simulink model "case4"  (R2024b)
settings: Solver=FixedStepAuto  StartTime=0  StopTime=1  FixedStep=1e-7  RelTol=1e-3
values from neighbouring files (symbols this model uses):
  SG_D_1_D = 0.01056    [IEEE9_case_parameters.m]    (also in case1_parameters.m; case2_parameters.m; case3_parameters.m; case4_parameters.m)
  SG_D_1_EnableSaturation = 0    [IEEE9_case_parameters.m]    (also in case1_parameters.m; case2_parameters.m; case3_parameters.m; case4_parameters.m)
  SG_D_1_f0 = 60    [IEEE9_case_parameters.m]    (also in case1_parameters.m; case2_parameters.m; case3_parameters.m; case4_parameters.m)
  SG_D_1_H = 7.5    [IEEE9_case_parameters.m]    (also in case1_parameters.m; case2_parameters.m; case3_parameters.m; case4_parameters.m)
  SG_D_1_K_A = 20    [IEEE9_case_parameters.m]    (also in case1_parameters.m; case2_parameters.m; case3_parameters.m; case4_parameters.m)
  SG_D_1_K_E = 1.000000e+1    (= 10)    [IEEE9_case_parameters.m]    (also in case1_parameters.m; case2_parameters.m; case3_parameters.m; case4_parameters.m)
  SG_D_1_K_F = 2.363    [IEEE9_case_parameters.m]    (also in case1_parameters.m; case2_parameters.m; case3_parameters.m; case4_parameters.m)
  SG_D_1_K_s = 0.5    [IEEE9_case_parameters.m]    (also in case1_parameters.m = 5; case2_parameters.m = 5; case3_parameters.m = 5; case4_parameters.m = 5)
  SG_D_1_R_a = 0.001088    [IEEE9_case_parameters.m]    (also in case1_parameters.m; case2_parameters.m; case3_parameters.m; case4_parameters.m)
  SG_D_1_S_A = 1    [IEEE9_case_parameters.m]    (also in case1_parameters.m; case2_parameters.m; case3_parameters.m; case4_parameters.m)
  SG_D_1_S_B = 0.103    [IEEE9_case_parameters.m]    (also in case1_parameters.m; case2_parameters.m; case3_parameters.m; case4_parameters.m)
  SG_D_1_S_N = 10.659857    [IEEE9_case_parameters.m]    (also in case1_parameters.m; case2_parameters.m; case3_parameters.m; case4_parameters.m)
  SG_D_1_SpeedPara = 200    [IEEE9_case_parameters.m]    (also in case1_parameters.m; case2_parameters.m; case3_parameters.m; case4_parameters.m)
  SG_D_1_T_0 = 0.720173    [IEEE9_case_parameters.m]    (also in case1_parameters.m = 0.755522; case2_parameters.m = 0.808931; case3_parameters.m = 0.869402; case4_parameters.m = 0.729316)
  SG_D_1_T_1 = 0.3    [IEEE9_case_parameters.m]    (also in case1_parameters.m; case2_parameters.m; case3_parameters.m; case4_parameters.m)
  SG_D_1_T_2 = 0.05    [IEEE9_case_parameters.m]    (also in case1_parameters.m; case2_parameters.m; case3_parameters.m; case4_parameters.m)
  SG_D_1_T_3 = 0.02    [IEEE9_case_parameters.m]    (also in case1_parameters.m; case2_parameters.m; case3_parameters.m; case4_parameters.m)
  SG_D_1_T_4 = 0.005    [IEEE9_case_parameters.m]    (also in case1_parameters.m; case2_parameters.m; case3_parameters.m; case4_parameters.m)
  SG_D_1_T_A = 0.02    [IEEE9_case_parameters.m]    (also in case1_parameters.m; case2_parameters.m; case3_parameters.m; case4_parameters.m)
  SG_D_1_T_dd = 8.000000e+0    (= 8)    [IEEE9_case_parameters.m]    (also in case1_parameters.m; case2_parameters.m; case3_parameters.m; case4_parameters.m)
  SG_D_1_T_ddd = 0.04    [IEEE9_case_parameters.m]    (also in case1_parameters.m; case2_parameters.m; case3_parameters.m; case4_parameters.m)
  SG_D_1_T_E = 0.314    [IEEE9_case_parameters.m]    (also in case1_parameters.m; case2_parameters.m; case3_parameters.m; case4_parameters.m)
  SG_D_1_T_F = 0.35    [IEEE9_case_parameters.m]    (also in case1_parameters.m; case2_parameters.m; case3_parameters.m; case4_parameters.m)
  SG_D_1_T_qd = 0.8    [IEEE9_case_parameters.m]    (also in case1_parameters.m; case2_parameters.m; case3_parameters.m; case4_parameters.m)
  SG_D_1_T_qdd = 0.02    [IEEE9_case_parameters.m]    (also in case1_parameters.m; case2_parameters.m; case3_parameters.m; case4_parameters.m)
  SG_D_1_T_speed = 0.1    [IEEE9_case_parameters.m]    (also in case1_parameters.m = 200; case2_parameters.m = 200; case3_parameters.m = 200; case4_parameters.m = 200)
  SG_D_1_T_w = 0.5    [IEEE9_case_parameters.m]    (also in case1_parameters.m; case2_parameters.m; case3_parameters.m; case4_parameters.m)
  SG_D_1_V_ref = 1.990276    [IEEE9_case_parameters.m]    (also in case1_parameters.m = 2.042296; case2_parameters.m = 2.051388; case3_parameters.m = 2.089584; case4_parameters.m = 2.01845)
  SG_D_1_w_ref = 376.991118    [IEEE9_case_parameters.m]    (also in case1_parameters.m; case2_parameters.m; case3_parameters.m; case4_parameters.m)
  SG_D_1_wb = 6.000000e+1    (= 60)    [IEEE9_case_parameters.m]    (also in case1_parameters.m; case2_parameters.m; case3_parameters.m; case4_parameters.m)
  SG_D_1_x_d = 1.9    [IEEE9_case_parameters.m]    (also in case1_parameters.m; case2_parameters.m; case3_parameters.m; case4_parameters.m)
  SG_D_1_x_dd = 0.302    [IEEE9_case_parameters.m]    (also in case1_parameters.m; case2_parameters.m; case3_parameters.m; case4_parameters.m)
  SG_D_1_x_ddd = 0.204    [IEEE9_case_parameters.m]    (also in case1_parameters.m; case2_parameters.m; case3_parameters.m; case4_parameters.m)
  SG_D_1_x_l = 0.05    [IEEE9_case_parameters.m]    (also in case1_parameters.m; case2_parameters.m; case3_parameters.m; case4_parameters.m)
  SG_D_1_x_q = 1.3    [IEEE9_case_parameters.m]    (also in case1_parameters.m; case2_parameters.m; case3_parameters.m; case4_parameters.m)
  SG_D_1_x_qd = 0.5    [IEEE9_case_parameters.m]    (also in case1_parameters.m; case2_parameters.m; case3_parameters.m; case4_parameters.m)
  SG_D_1_x_qdd = 0.3    [IEEE9_case_parameters.m]    (also in case1_parameters.m; case2_parameters.m; case3_parameters.m; case4_parameters.m)
  SG_D_2_D = 0.02    [IEEE9_case_parameters.m]    (also in case1_parameters.m; case2_parameters.m; case3_parameters.m; case4_parameters.m)
  SG_D_2_EnableSaturation = 0    [IEEE9_case_parameters.m]    (also in case1_parameters.m; case2_parameters.m; case3_parameters.m; case4_parameters.m)
  SG_D_2_f0 = 60    [IEEE9_case_parameters.m]    (also in case1_parameters.m; case2_parameters.m; case3_parameters.m; case4_parameters.m)
  SG_D_2_H = 8.000000e+0    (= 8)    [IEEE9_case_parameters.m]    (also in case1_parameters.m; case2_parameters.m; case3_parameters.m; case4_parameters.m)
  SG_D_2_K_A = 20    [IEEE9_case_parameters.m]    (also in case1_parameters.m; case2_parameters.m; case3_parameters.m; case4_parameters.m)
  SG_D_2_K_E = 1.000000e+1    (= 10)    [IEEE9_case_parameters.m]    (also in case1_parameters.m; case2_parameters.m; case3_parameters.m; case4_parameters.m)
  SG_D_2_K_F = 2.363    [IEEE9_case_parameters.m]    (also in case1_parameters.m; case2_parameters.m; case3_parameters.m; case4_parameters.m)
  SG_D_2_K_s = 0.5    [IEEE9_case_parameters.m]    (also in case1_parameters.m = 4; case2_parameters.m = 4; case3_parameters.m = 4; case4_parameters.m = 4)
  SG_D_2_R_a = 0.001088    [IEEE9_case_parameters.m]    (also in case1_parameters.m; case2_parameters.m; case3_parameters.m; case4_parameters.m)
  SG_D_2_S_A = 1    [IEEE9_case_parameters.m]    (also in case1_parameters.m; case2_parameters.m; case3_parameters.m; case4_parameters.m)
  SG_D_2_S_B = 0.103    [IEEE9_case_parameters.m]    (also in case1_parameters.m; case2_parameters.m; case3_parameters.m; case4_parameters.m)
  SG_D_2_S_N = 10.659857    [IEEE9_case_parameters.m]    (also in case1_parameters.m; case2_parameters.m; case3_parameters.m; case4_parameters.m)
  SG_D_2_SpeedPara = 200    [IEEE9_case_parameters.m]    (also in case1_parameters.m; case2_parameters.m; case3_parameters.m; case4_parameters.m)
  SG_D_2_T_0 = 1.632913    [IEEE9_case_parameters.m]    (also in case1_parameters.m = 1.632925; case2_parameters.m = 1.632915; case3_parameters.m = 1.632914; case4_parameters.m = 1.632927)
  SG_D_2_T_1 = 0.2    [IEEE9_case_parameters.m]    (also in case1_parameters.m; case2_parameters.m; case3_parameters.m; case4_parameters.m)
  SG_D_2_T_2 = 0.05    [IEEE9_case_parameters.m]    (also in case1_parameters.m; case2_parameters.m; case3_parameters.m; case4_parameters.m)
  SG_D_2_T_3 = 0.02    [IEEE9_case_parameters.m]    (also in case1_parameters.m; case2_parameters.m; case3_parameters.m; case4_parameters.m)
  SG_D_2_T_4 = 0.005    [IEEE9_case_parameters.m]    (also in case1_parameters.m; case2_parameters.m; case3_parameters.m; case4_parameters.m)
  SG_D_2_T_A = 0.02    [IEEE9_case_parameters.m]    (also in case1_parameters.m; case2_parameters.m; case3_parameters.m; case4_parameters.m)
  SG_D_2_T_dd = 7.9    [IEEE9_case_parameters.m]    (also in case1_parameters.m; case2_parameters.m; case3_parameters.m; case4_parameters.m)
  SG_D_2_T_ddd = 0.04    [IEEE9_case_parameters.m]    (also in case1_parameters.m; case2_parameters.m; case3_parameters.m; case4_parameters.m)
  SG_D_2_T_E = 0.314    [IEEE9_case_parameters.m]    (also in case1_parameters.m; case2_parameters.m; case3_parameters.m; case4_parameters.m)
  SG_D_2_T_F = 0.35    [IEEE9_case_parameters.m]    (also in case1_parameters.m; case2_parameters.m; case3_parameters.m; case4_parameters.m)
  SG_D_2_T_qd = 0.8    [IEEE9_case_parameters.m]    (also in case1_parameters.m; case2_parameters.m; case3_parameters.m; case4_parameters.m)
  SG_D_2_T_qdd = 0.015    [IEEE9_case_parameters.m]    (also in case1_parameters.m; case2_parameters.m; case3_parameters.m; case4_parameters.m)
  SG_D_2_T_speed = 0.1    [IEEE9_case_parameters.m]    (also in case1_parameters.m = 150; case2_parameters.m = 150; case3_parameters.m = 150; case4_parameters.m = 150)
  SG_D_2_T_w = 0.35    [IEEE9_case_parameters.m]    (also in case1_parameters.m; case2_parameters.m; case3_parameters.m; case4_parameters.m)
  SG_D_2_V_ref = 2.58547    [IEEE9_case_parameters.m]    (also in case1_parameters.m = 2.597896; case2_parameters.m = 2.587136; case3_parameters.m = 2.586042; case4_parameters.m = 2.599679)
  SG_D_2_w_ref = 376.991118    [IEEE9_case_parameters.m]    (also in case1_parameters.m; case2_parameters.m; case3_parameters.m; case4_parameters.m)
  SG_D_2_wb = 6.000000e+1    (= 60)    [IEEE9_case_parameters.m]    (also in case1_parameters.m; case2_parameters.m; case3_parameters.m; case4_parameters.m)
  SG_D_2_x_d = 1.8    [IEEE9_case_parameters.m]    (also in case1_parameters.m; case2_parameters.m; case3_parameters.m; case4_parameters.m)
  SG_D_2_x_dd = 0.302    [IEEE9_case_parameters.m]    (also in case1_parameters.m; case2_parameters.m; case3_parameters.m; case4_parameters.m)
  SG_D_2_x_ddd = 0.204    [IEEE9_case_parameters.m]    (also in case1_parameters.m; case2_parameters.m; case3_parameters.m; case4_parameters.m)
  SG_D_2_x_l = 0.05    [IEEE9_case_parameters.m]    (also in case1_parameters.m; case2_parameters.m; case3_parameters.m; case4_parameters.m)
  SG_D_2_x_q = 1.25    [IEEE9_case_parameters.m]    (also in case1_parameters.m; case2_parameters.m; case3_parameters.m; case4_parameters.m)
  SG_D_2_x_qd = 0.5    [IEEE9_case_parameters.m]    (also in case1_parameters.m; case2_parameters.m; case3_parameters.m; case4_parameters.m)
  SG_D_2_x_qdd = 0.3    [IEEE9_case_parameters.m]    (also in case1_parameters.m; case2_parameters.m; case3_parameters.m; case4_parameters.m)
  SG_D_3_D = 0.02    [IEEE9_case_parameters.m]    (also in case1_parameters.m; case2_parameters.m; case3_parameters.m; case4_parameters.m)
  SG_D_3_EnableSaturation = 0    [IEEE9_case_parameters.m]    (also in case1_parameters.m; case2_parameters.m; case3_parameters.m; case4_parameters.m)
  SG_D_3_f0 = 60    [IEEE9_case_parameters.m]    (also in case1_parameters.m; case2_parameters.m; case3_parameters.m; case4_parameters.m)
  SG_D_3_H = 7.7    [IEEE9_case_parameters.m]    (also in case1_parameters.m; case2_parameters.m; case3_parameters.m; case4_parameters.m)
  SG_D_3_K_A = 20    [IEEE9_case_parameters.m]    (also in case1_parameters.m; case2_parameters.m; case3_parameters.m; case4_parameters.m)
  SG_D_3_K_E = 1.000000e+1    (= 10)    [IEEE9_case_parameters.m]    (also in case1_parameters.m; case2_parameters.m; case3_parameters.m; case4_parameters.m)
  SG_D_3_K_F = 2.363    [IEEE9_case_parameters.m]    (also in case1_parameters.m; case2_parameters.m; case3_parameters.m; case4_parameters.m)
  SG_D_3_K_s = 0.2    [IEEE9_case_parameters.m]    (also in case1_parameters.m = 2; case2_parameters.m = 2; case3_parameters.m = 2; case4_parameters.m = 2)
  SG_D_3_R_a = 0.001088    [IEEE9_case_parameters.m]    (also in case1_parameters.m; case2_parameters.m; case3_parameters.m; case4_parameters.m)
  SG_D_3_S_A = 1    [IEEE9_case_parameters.m]    (also in case1_parameters.m; case2_parameters.m; case3_parameters.m; case4_parameters.m)
  SG_D_3_S_B = 0.103    [IEEE9_case_parameters.m]    (also in case1_parameters.m; case2_parameters.m; case3_parameters.m; case4_parameters.m)
  SG_D_3_S_N = 10.659857    [IEEE9_case_parameters.m]    (also in case1_parameters.m; case2_parameters.m; case3_parameters.m; case4_parameters.m)
  SG_D_3_SpeedPara = 200    [IEEE9_case_parameters.m]    (also in case1_parameters.m; case2_parameters.m; case3_parameters.m; case4_parameters.m)
  SG_D_3_T_0 = 0.850788    [IEEE9_case_parameters.m]    (also in case1_parameters.m = 0.850786; case2_parameters.m = 0.850787; case3_parameters.m; case4_parameters.m = 0.850786)
  SG_D_3_T_1 = 0.2    [IEEE9_case_parameters.m]    (also in case1_parameters.m; case2_parameters.m; case3_parameters.m; case4_parameters.m)
  SG_D_3_T_2 = 0.05    [IEEE9_case_parameters.m]    (also in case1_parameters.m; case2_parameters.m; case3_parameters.m; case4_parameters.m)
  SG_D_3_T_3 = 0.02    [IEEE9_case_parameters.m]    (also in case1_parameters.m; case2_parameters.m; case3_parameters.m; case4_parameters.m)
  SG_D_3_T_4 = 0.005    [IEEE9_case_parameters.m]    (also in case1_parameters.m; case2_parameters.m; case3_parameters.m; case4_parameters.m)
  SG_D_3_T_A = 0.02    [IEEE9_case_parameters.m]    (also in case1_parameters.m; case2_parameters.m; case3_parameters.m; case4_parameters.m)
  SG_D_3_T_dd = 8.1    [IEEE9_case_parameters.m]    (also in case1_parameters.m; case2_parameters.m; case3_parameters.m; case4_parameters.m)
  SG_D_3_T_ddd = 0.04    [IEEE9_case_parameters.m]    (also in case1_parameters.m; case2_parameters.m; case3_parameters.m; case4_parameters.m)
  SG_D_3_T_E = 0.314    [IEEE9_case_parameters.m]    (also in case1_parameters.m; case2_parameters.m; case3_parameters.m; case4_parameters.m)
  SG_D_3_T_F = 0.35    [IEEE9_case_parameters.m]    (also in case1_parameters.m; case2_parameters.m; case3_parameters.m; case4_parameters.m)
  SG_D_3_T_qd = 0.8    [IEEE9_case_parameters.m]    (also in case1_parameters.m; case2_parameters.m; case3_parameters.m; case4_parameters.m)
  SG_D_3_T_qdd = 0.015    [IEEE9_case_parameters.m]    (also in case1_parameters.m; case2_parameters.m; case3_parameters.m; case4_parameters.m)
  SG_D_3_T_speed = 0.1    [IEEE9_case_parameters.m]    (also in case1_parameters.m = 180; case2_parameters.m = 180; case3_parameters.m = 180; case4_parameters.m = 180)
  SG_D_3_T_w = 0.4    [IEEE9_case_parameters.m]    (also in case1_parameters.m; case2_parameters.m; case3_parameters.m; case4_parameters.m)
  SG_D_3_V_ref = 1.892727    [IEEE9_case_parameters.m]    (also in case1_parameters.m = 1.906439; case2_parameters.m = 1.895535; case3_parameters.m = 1.892105; case4_parameters.m = 1.906598)
  SG_D_3_w_ref = 376.991118    [IEEE9_case_parameters.m]    (also in case1_parameters.m; case2_parameters.m; case3_parameters.m; case4_parameters.m)
  SG_D_3_wb = 6.000000e+1    (= 60)    [IEEE9_case_parameters.m]    (also in case1_parameters.m; case2_parameters.m; case3_parameters.m; case4_parameters.m)
  SG_D_3_x_d = 1.85    [IEEE9_case_parameters.m]    (also in case1_parameters.m; case2_parameters.m; case3_parameters.m; case4_parameters.m)
  SG_D_3_x_dd = 0.302    [IEEE9_case_parameters.m]    (also in case1_parameters.m; case2_parameters.m; case3_parameters.m; case4_parameters.m)
  SG_D_3_x_ddd = 0.204    [IEEE9_case_parameters.m]    (also in case1_parameters.m; case2_parameters.m; case3_parameters.m; case4_parameters.m)
  SG_D_3_x_l = 0.05    [IEEE9_case_parameters.m]    (also in case1_parameters.m; case2_parameters.m; case3_parameters.m; case4_parameters.m)
  SG_D_3_x_q = 1.2    [IEEE9_case_parameters.m]    (also in case1_parameters.m; case2_parameters.m; case3_parameters.m; case4_parameters.m)
  SG_D_3_x_qd = 0.5    [IEEE9_case_parameters.m]    (also in case1_parameters.m; case2_parameters.m; case3_parameters.m; case4_parameters.m)
  SG_D_3_x_qdd = 0.3    [IEEE9_case_parameters.m]    (also in case1_parameters.m; case2_parameters.m; case3_parameters.m; case4_parameters.m)
(part 8 of 12)

== system case4/SG_D_2/d_psi_d_SG_D_2_block ==
  note: d_psi_d_SG_D_2 in case4
      | $2\,\pi \,f_{0}\,\left(v_{d,\mathrm{SG},D,2}\,\sin\left(\theta _{\mathrm{SG},D,2}\right)-v_{q,\mathrm{SG},D,2}\,\cos\left(\theta _{\mathrm{SG},D,2}\right)+\frac{R_{a}\,\left(\frac{\psi _{\mathrm{1d},\mathrm{SG},D,2}\,\left(x_{\mathrm{dd}}-x_{\mathrm{ddd}}\right)}{x_{\mathrm{dd}}-x_{l}}-\psi _{d,\mathrm{SG},D,2}+\frac{\psi _{\mathrm{fd},\mathrm{SG},D,2}\,\left(x_{\mathrm{ddd}}-x_{l}\right)}{x_{\mathrm{dd}}-x_{l}}\right)}{x_{\mathrm{ddd}}}+\frac{\psi _{q,\mathrm{SG},D,2}\,w_{\mathrm{SG},D,2}}{2\,f_{0}\,\pi }\right)$
      | Automatically generated on 2025-10-31 19:05:14 .
  State_psi_1d_SG_D_2_e94c1 : Inport
  State_psi_d_SG_D_2_af81e : Inport  Port=2
  State_psi_fd_SG_D_2_c88a6 : Inport  Port=3
  Input_v_d_SG_D_2_dee58 : Inport  Port=4
  State_theta_SG_D_2_f56a2 : Inport  Port=5
  Input_v_q_SG_D_2_fe918 : Inport  Port=6
  State_theta_SG_D_2_7f4d5 : Inport  Port=7
  State_psi_q_SG_D_2_4ef81 : Inport  Port=8
  State_w_SG_D_2_062a2 : Inport  Port=9
  Add_59c16 : Sum
  Add_65186 : Sum
  Constant_-1_036a7 : Constant  Value=-1
  Constant_-2.0_3973c : Constant  Value=-2.0
  Constant_2.0_6257b : Constant  Value=2.0
  Constant_R_a_b919b : Constant  Value=R_a
  Constant_f0_3cef4 : Constant  Value=f0
  Constant_f0_d0e35 : Constant  Value=f0
  Constant_pi_2f3ee : Constant  Value=pi
  Constant_pi_37ca9 : Constant  Value=pi
  Constant_x_dd_3da7b : Constant  Value=x_dd
  Constant_x_dd_8e33d : Constant  Value=x_dd
  Constant_x_dd_ba832 : Constant  Value=x_dd
  Constant_x_ddd_7c835 : Constant  Value=x_ddd
  Constant_x_ddd_7e8dd : Constant  Value=x_ddd
  Constant_x_ddd_e232c : Constant  Value=x_ddd
  Constant_x_l_d0b80 : Constant  Value=x_l
  Constant_x_l_e7e86 : Constant  Value=x_l
  Constant_x_l_ffaeb : Constant  Value=x_l
  Divide_76b6b : Product  Inputs=*/
  Divide_b3d15 : Product  Inputs=*/
  Divide_b777e : Product  Inputs=*/
  Divide_e2439 : Product  Inputs=*/
  MathFunc_cos_4ccf5 : Trigonometry  Operator=cos
  MathFunc_sin_3f72b : Trigonometry
  Product_03847 : Product
  Product_0ac18 : Product
  Product_38d7c : Product
  Product_61013 : Product
  Product_9d298 : Product
  Product_9e494 : Product
  Product_aa42e : Product
  Product_b53b5 : Product
  Product_c12d3 : Product
  Product_c215c : Product
  Product_e705f : Product
  Product_f92ad : Product
  Subtract_020bf : Sum  Inputs=+-
  Subtract_1fd1b : Sum  Inputs=+-
  Subtract_3097e : Sum  Inputs=+-
  Subtract_37338 : Sum  Inputs=+-
  Subtract_37bb0 : Sum  Inputs=+-
  Subtract_7214a : Sum  Inputs=+-
  Subtract_b4a33 : Sum  Inputs=+-
  Blockout_d_psi_d_SG_D_2_f1be8 : Outport
  wires:
  MathFunc_sin_3f72b/1 -> Product_03847/2
  Constant_x_dd_3da7b/1 -> Subtract_37bb0/1
  Constant_-1_036a7/1 -> Product_b53b5/1
  Constant_x_l_d0b80/1 -> Subtract_37bb0/2
  State_psi_1d_SG_D_2_e94c1/1 -> Product_b53b5/2
  Constant_f0_3cef4/1 -> Product_9e494/2
  Constant_2.0_6257b/1 -> Product_c215c/1
  Constant_x_l_ffaeb/1 -> Subtract_020bf/2
  Constant_x_dd_8e33d/1 -> Subtract_3097e/1
  Product_38d7c/1 -> Blockout_d_psi_d_SG_D_2_f1be8/1
  Constant_pi_2f3ee/1 -> Product_c215c/2
  Constant_x_ddd_7c835/1 -> Subtract_3097e/2
  Subtract_37338/1 -> Product_38d7c/2
  Product_b53b5/1 -> Product_e705f/1
  Product_c215c/1 -> Product_9d298/1
  Subtract_3097e/1 -> Product_e705f/2
  Divide_b3d15/1 -> Subtract_37338/2
  Constant_x_ddd_7e8dd/1 -> Subtract_7214a/1
  Constant_x_l_e7e86/1 -> Subtract_7214a/2
  Product_e705f/1 -> Divide_e2439/1
  Subtract_b4a33/1 -> Add_59c16/1
  Subtract_37bb0/1 -> Divide_e2439/2
  State_psi_fd_SG_D_2_c88a6/1 -> Product_aa42e/1
  Subtract_7214a/1 -> Product_aa42e/2
  Constant_x_dd_ba832/1 -> Subtract_020bf/1
  Divide_e2439/1 -> Add_65186/1
  State_psi_d_SG_D_2_af81e/1 -> Add_65186/2
  Product_aa42e/1 -> Divide_76b6b/1
  Subtract_020bf/1 -> Divide_76b6b/2
  Add_65186/1 -> Subtract_1fd1b/1
  Divide_76b6b/1 -> Subtract_1fd1b/2
  Constant_R_a_b919b/1 -> Product_c12d3/1
  Subtract_1fd1b/1 -> Product_c12d3/2
  Divide_b777e/1 -> Subtract_b4a33/1
  State_theta_SG_D_2_f56a2/1 -> MathFunc_sin_3f72b/1
  Product_c12d3/1 -> Divide_b777e/1
  Constant_-2.0_3973c/1 -> Product_0ac18/1
  Input_v_d_SG_D_2_dee58/1 -> Product_03847/1
  Constant_x_ddd_e232c/1 -> Divide_b777e/2
  State_theta_SG_D_2_7f4d5/1 -> MathFunc_cos_4ccf5/1
  Product_9e494/1 -> Product_38d7c/1
  Product_03847/1 -> Subtract_b4a33/2
  Product_0ac18/1 -> Product_9e494/1
  Input_v_q_SG_D_2_fe918/1 -> Product_61013/1
  MathFunc_cos_4ccf5/1 -> Product_61013/2
  State_psi_q_SG_D_2_4ef81/1 -> Product_f92ad/1
  State_w_SG_D_2_062a2/1 -> Product_f92ad/2
  Constant_f0_d0e35/1 -> Product_9d298/2
  Constant_pi_37ca9/1 -> Product_0ac18/2
  Product_61013/1 -> Add_59c16/2
  Product_f92ad/1 -> Divide_b3d15/1
  Product_9d298/1 -> Divide_b3d15/2
  Add_59c16/1 -> Subtract_37338/1

== system case4/SG_D_2/d_psi_fd_SG_D_2_block ==
  note: d_psi_fd_SG_D_2 in case4
      | $-\frac{\psi _{\mathrm{fd},\mathrm{SG},D,2}-E_{\mathrm{fd},\mathrm{SG},D,2}+\left(x_{d}-x_{\mathrm{dd}}\right)\,\left(\frac{\frac{\psi _{\mathrm{1d},\mathrm{SG},D,2}\,\left(x_{\mathrm{dd}}-x_{\mathrm{ddd}}\right)}{x_{\mathrm{dd}}-x_{l}}-\psi _{d,\mathrm{SG},D,2}+\frac{\psi _{\mathrm{fd},\mathrm{SG},D,2}\,\left(x_{\mathrm{ddd}}-x_{l}\right)}{x_{\mathrm{dd}}-x_{l}}}{x_{\mathrm{ddd}}}-\frac{\left(x_{\mathrm{dd}}-x_{\mathrm{ddd}}\right)\,\left(\psi _{\mathrm{1d},\mathrm{SG},D,2}-\psi _{\mathrm{fd},\mathrm{SG},D,2}+\frac{\left(x_{\mathrm{dd}}-x_{l}\right)\,\left(\frac{\psi _{\mathrm{1d},\mathrm{SG},D,2}\,\left(x_{\mathrm{dd}}-x_{\mathrm{ddd}}\right)}{x_{\mathrm{dd}}-x_{l}}-\psi _{d,\mathrm{SG},D,2}+\frac{\psi _{\mathrm{fd},\mathrm{SG},D,2}\,\left(x_{\mathrm{ddd}}-x_{l}\right)}{x_{\mathrm{dd}}-x_{l}}\right)}{x_{\mathrm{ddd}}}\right)}{{\left(x_{\mathrm{dd}}-x_{l}\right)}^2}\right)}{T_{\mathrm{dd}}}$
      | Automatically generated on 2025-10-31 19:05:22 .
  State_E_fd_SG_D_2_f08a6 : Inport
  State_psi_fd_SG_D_2_402f0 : Inport  Port=2
  State_psi_1d_SG_D_2_343a2 : Inport  Port=3
  State_psi_fd_SG_D_2_f381f : Inport  Port=4
  State_psi_1d_SG_D_2_7e680 : Inport  Port=5
  State_psi_d_SG_D_2_a4384 : Inport  Port=6
  State_psi_fd_SG_D_2_f7400 : Inport  Port=7
  State_psi_1d_SG_D_2_84c2e : Inport  Port=8
  State_psi_d_SG_D_2_a1f54 : Inport  Port=9
  State_psi_fd_SG_D_2_88820 : Inport  Port=10
  Add_90f4d : Sum
  Add_c59e4 : Sum
  Constant_-1_72afa : Constant  Value=-1
  Constant_-1_7fc96 : Constant  Value=-1
  Constant_-1_ba4d7 : Constant  Value=-1
  Constant_2.0_47b63 : Constant  Value=2.0
  Constant_T_dd_95f7f : Constant  Value=T_dd
  Constant_x_d_f6139 : Constant  Value=x_d
  Constant_x_dd_1aaad : Constant  Value=x_dd
  Constant_x_dd_21c19 : Constant  Value=x_dd
  Constant_x_dd_332b4 : Constant  Value=x_dd
  Constant_x_dd_46b3b : Constant  Value=x_dd
  Constant_x_dd_46ef8 : Constant  Value=x_dd
  Constant_x_dd_4a258 : Constant  Value=x_dd
  Constant_x_dd_7c034 : Constant  Value=x_dd
  Constant_x_dd_c8e65 : Constant  Value=x_dd
  Constant_x_dd_d957f : Constant  Value=x_dd
  Constant_x_dd_efaec : Constant  Value=x_dd
  Constant_x_ddd_0397c : Constant  Value=x_ddd
  Constant_x_ddd_230ef : Constant  Value=x_ddd
  Constant_x_ddd_38a8f : Constant  Value=x_ddd
  Constant_x_ddd_3aa21 : Constant  Value=x_ddd
  Constant_x_ddd_4aca7 : Constant  Value=x_ddd
  Constant_x_ddd_cc4cb : Constant  Value=x_ddd
  Constant_x_ddd_e90fc : Constant  Value=x_ddd
  Constant_x_l_01d2d : Constant  Value=x_l
  Constant_x_l_0c75b : Constant  Value=x_l
  Constant_x_l_29d03 : Constant  Value=x_l
  Constant_x_l_668a6 : Constant  Value=x_l
  Constant_x_l_88bfb : Constant  Value=x_l
  Constant_x_l_a3b0a : Constant  Value=x_l
  Constant_x_l_ab383 : Constant  Value=x_l
  Constant_x_l_dfccb : Constant  Value=x_l
  Divide_5dc04 : Product  Inputs=*/
  Divide_74695 : Product  Inputs=*/
  Divide_86339 : Product  Inputs=*/
  Divide_a3082 : Product  Inputs=*/
  Divide_a8f56 : Product  Inputs=*/
  Divide_c07df : Product  Inputs=*/
  Divide_cb102 : Product  Inputs=*/
  Divide_d3bd8 : Product  Inputs=*/
  Power_8abed : Math  Operator=pow
  Product_304fb : Product
  Product_4cb9f : Product
  Product_6624d : Product
  Product_6677c : Product
  Product_80e23 : Product
  Product_a36e0 : Product
  Product_b882c : Product
  Product_ba160 : Product
  Product_c7ca2 : Product
  Product_e1148 : Product
  Subtract_23522 : Sum  Inputs=+-
  Subtract_29169 : Sum  Inputs=+-
  Subtract_317c3 : Sum  Inputs=+-
  Subtract_4a274 : Sum  Inputs=+-
  Subtract_4e9bf : Sum  Inputs=+-
  Subtract_75da6 : Sum  Inputs=+-
  Subtract_82e0a : Sum  Inputs=+-
  Subtract_89ded : Sum  Inputs=+-
  Subtract_9c655 : Sum  Inputs=+-
  Subtract_adbdf : Sum  Inputs=+-
  Subtract_bb221 : Sum  Inputs=+-
  Subtract_c75bf : Sum  Inputs=+-
  Subtract_cc98b : Sum  Inputs=+-
  Subtract_ccf6c : Sum  Inputs=+-
  Subtract_cde66 : Sum  Inputs=+-
  Subtract_ddcae : Sum  Inputs=+-
  Subtract_e443b : Sum  Inputs=+-
  Subtract_e7b0c : Sum  Inputs=+-
  Subtract_f28af : Sum  Inputs=+-
  Blockout_d_psi_fd_SG_D_2_9880d : Outport
  wires:
  Constant_x_dd_21c19/1 -> Subtract_89ded/1
  Constant_-1_ba4d7/1 -> Product_4cb9f/1
  Constant_x_l_0c75b/1 -> Subtract_317c3/2
  Divide_5dc04/1 -> Add_c59e4/1
  Subtract_29169/1 -> Product_6624d/2
  Constant_x_l_a3b0a/1 -> Subtract_89ded/2
  Product_6624d/1 -> Divide_a8f56/1
  State_psi_1d_SG_D_2_7e680/1 -> Product_4cb9f/2
  Constant_x_dd_efaec/1 -> Subtract_c75bf/1
  Product_ba160/1 -> Divide_5dc04/1
  Constant_x_dd_332b4/1 -> Subtract_4a274/1
  Constant_x_ddd_230ef/1 -> Subtract_c75bf/2
  Constant_x_dd_46b3b/1 -> Subtract_cc98b/1
  Product_4cb9f/1 -> Product_c7ca2/1
  Subtract_c75bf/1 -> Product_c7ca2/2
  State_psi_d_SG_D_2_a1f54/1 -> Add_c59e4/2
  Constant_x_ddd_4aca7/1 -> Subtract_29169/1
  Constant_x_l_29d03/1 -> Subtract_29169/2
  Product_c7ca2/1 -> Divide_a3082/1
  Subtract_89ded/1 -> Divide_a3082/2
  State_psi_fd_SG_D_2_f7400/1 -> Product_6624d/1
  Subtract_ccf6c/1 -> Product_304fb/2
  Constant_x_dd_1aaad/1 -> Subtract_adbdf/1
  Constant_x_l_ab383/1 -> Subtract_adbdf/2
  Product_e1148/1 -> Product_304fb/1
  Divide_a3082/1 -> Add_90f4d/1
  State_psi_d_SG_D_2_a4384/1 -> Add_90f4d/2
  Subtract_adbdf/1 -> Divide_a8f56/2
  Constant_x_dd_7c034/1 -> Subtract_317c3/1
  Constant_x_ddd_3aa21/1 -> Subtract_75da6/1
  Add_90f4d/1 -> Subtract_cde66/1
  Divide_a8f56/1 -> Subtract_cde66/2
  Constant_-1_7fc96/1 -> Product_a36e0/1
  Product_80e23/1 -> Divide_cb102/1
  State_psi_1d_SG_D_2_84c2e/1 -> Product_a36e0/2
  Subtract_4a274/1 -> Product_e1148/2
  Constant_x_dd_d957f/1 -> Subtract_4e9bf/1
  Divide_cb102/1 -> Subtract_e443b/2
  Constant_-1_72afa/1 -> Product_e1148/1
  Constant_x_ddd_e90fc/1 -> Subtract_4e9bf/2
  Constant_x_ddd_0397c/1 -> Divide_86339/2
  Subtract_317c3/1 -> Product_b882c/1
  Subtract_cde66/1 -> Product_b882c/2
  State_psi_fd_SG_D_2_f381f/1 -> Subtract_f28af/2
  Product_a36e0/1 -> Product_ba160/1
  Subtract_4e9bf/1 -> Product_ba160/2
  Constant_2.0_47b63/1 -> Power_8abed/2
  State_psi_1d_SG_D_2_343a2/1 -> Subtract_f28af/1
  Constant_x_dd_4a258/1 -> Subtract_82e0a/1
  Subtract_75da6/1 -> Product_80e23/2
  Constant_x_l_668a6/1 -> Subtract_82e0a/2
  Constant_x_l_01d2d/1 -> Subtract_75da6/2
  Constant_x_ddd_cc4cb/1 -> Subtract_4a274/2
  Subtract_cc98b/1 -> Divide_cb102/2
  Product_b882c/1 -> Divide_86339/1
  Subtract_82e0a/1 -> Divide_5dc04/2
  State_psi_fd_SG_D_2_88820/1 -> Product_80e23/1
  Constant_x_l_dfccb/1 -> Subtract_cc98b/2
  Constant_x_dd_46ef8/1 -> Subtract_bb221/1
  Subtract_f28af/1 -> Subtract_ccf6c/1
  Divide_86339/1 -> Subtract_ccf6c/2
  Constant_x_l_88bfb/1 -> Subtract_bb221/2
  Subtract_bb221/1 -> Power_8abed/1
  Add_c59e4/1 -> Subtract_e443b/1
  Product_304fb/1 -> Divide_d3bd8/1
  Power_8abed/1 -> Divide_d3bd8/2
  Subtract_e443b/1 -> Divide_74695/1
  Constant_x_ddd_38a8f/1 -> Divide_74695/2
  Constant_x_d_f6139/1 -> Subtract_23522/1
  Constant_x_dd_c8e65/1 -> Subtract_23522/2
  Divide_d3bd8/1 -> Subtract_9c655/1
  Divide_74695/1 -> Subtract_9c655/2
  State_E_fd_SG_D_2_f08a6/1 -> Subtract_ddcae/1
  State_psi_fd_SG_D_2_402f0/1 -> Subtract_ddcae/2
  Subtract_23522/1 -> Product_6677c/1
  Subtract_9c655/1 -> Product_6677c/2
  Subtract_ddcae/1 -> Subtract_e7b0c/1
  Product_6677c/1 -> Subtract_e7b0c/2
  Subtract_e7b0c/1 -> Divide_c07df/1
  Constant_T_dd_95f7f/1 -> Divide_c07df/2
  Divide_c07df/1 -> Blockout_d_psi_fd_SG_D_2_9880d/1

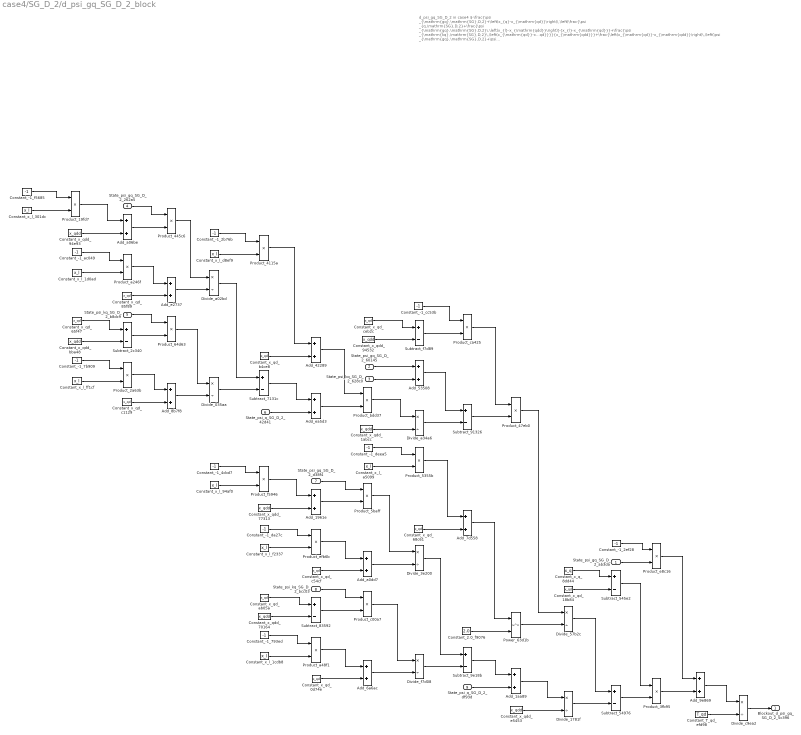
== system case4/SG_D_2/d_psi_gq_SG_D_2_block ==
  note: d_psi_gq_SG_D_2 in case4
      | $-\frac{\psi _{\mathrm{gq},\mathrm{SG},D,2}+\left(x_{q}-x_{\mathrm{qd}}\right)\,\left(\frac{\psi _{q,\mathrm{SG},D,2}+\frac{\psi _{\mathrm{gq},\mathrm{SG},D,2}\,\left(x_{l}-x_{\mathrm{qdd}}\right)}{x_{l}-x_{\mathrm{qd}}}+\frac{\psi _{\mathrm{kq},\mathrm{SG},D,2}\,\left(x_{\mathrm{qd}}-x_{\mathrm{qdd}}\right)}{x_{l}-x_{\mathrm{qd}}}}{x_{\mathrm{qdd}}}+\frac{\left(x_{\mathrm{qd}}-x_{\mathrm{qdd}}\right)\,\left(\psi _{\mathrm{gq},\mathrm{SG},D,2}+\psi _{\mathrm{kq},\mathrm{SG},D,2}+\frac{\left(x_{l}-x_{\mathrm{qd}}\right)\,\left(\psi _{q,\mathrm{SG},D,2}+\frac{\psi _{\mathrm{gq},\mathrm{SG},D,2}\,\left(x_{l}-x_{\mathrm{qdd}}\right)}{x_{l}-x_{\mathrm{qd}}}+\frac{\psi _{\mathrm{kq},\mathrm{SG},D,2}\,\left(x_{\mathrm{qd}}-x_{\mathrm{qdd}}\right)}{x_{l}-x_{\mathrm{qd}}}\right)}{x_{\mathrm{qdd}}}\right)}{{\left(x_{l}-x_{\mathrm{qd}}\right)}^2}\right)}{T_{\mathrm{qd}}}$
      | Automatically generated on 2025-10-31 19:05:30 .
  State_psi_gq_SG_D_2_ab3da : Inport
  State_psi_gq_SG_D_2_60145 : Inport  Port=2
  State_psi_kq_SG_D_2_628c0 : Inport  Port=3
  State_psi_gq_SG_D_2_262a5 : Inport  Port=4
  State_psi_kq_SG_D_2_b8dc9 : Inport  Port=5
  State_psi_q_SG_D_2_42d41 : Inport  Port=6
  State_psi_gq_SG_D_2_d38f4 : Inport  Port=7
  State_psi_kq_SG_D_2_bcc03 : Inport  Port=8
  State_psi_q_SG_D_2_df93d : Inport  Port=9
  Add_1961e : Sum
  Add_1aa89 : Sum
  Add_42289 : Sum
  Add_53508 : Sum
  Add_6a6ac : Sum
  Add_7d558 : Sum
  Add_8b7f8 : Sum
  Add_9e869 : Sum
  Add_a06be : Sum
  Add_a0dd7 : Sum
  Add_e2737 : Sum
  Add_ea5d3 : Sum
  Constant_-1_2b76b : Constant  Value=-1
  Constant_-1_2ef28 : Constant  Value=-1
  Constant_-1_4cbd7 : Constant  Value=-1
  Constant_-1_793ed : Constant  Value=-1
  Constant_-1_7b909 : Constant  Value=-1
  Constant_-1_ac049 : Constant  Value=-1
  Constant_-1_cc53b : Constant  Value=-1
  Constant_-1_da27c : Constant  Value=-1
  Constant_-1_deea5 : Constant  Value=-1
  Constant_-1_f5685 : Constant  Value=-1
  Constant_2.0_f9076 : Constant  Value=2.0
  Constant_T_qd_efd98 : Constant  Value=T_qd
  Constant_x_l_1cdb8 : Constant  Value=x_l
  Constant_x_l_1d0ad : Constant  Value=x_l
  Constant_x_l_301dc : Constant  Value=x_l
  Constant_x_l_94af0 : Constant  Value=x_l
  Constant_x_l_a5099 : Constant  Value=x_l
  Constant_x_l_d8ef9 : Constant  Value=x_l
  Constant_x_l_f2337 : Constant  Value=x_l
  Constant_x_l_ff1cf : Constant  Value=x_l
  Constant_x_q_8dd44 : Constant  Value=x_q
  Constant_x_qd_0d74e : Constant  Value=x_qd
  Constant_x_qd_18b84 : Constant  Value=x_qd
  Constant_x_qd_65f47 : Constant  Value=x_qd
  Constant_x_qd_68c61 : Constant  Value=x_qd
  Constant_x_qd_85f89 : Constant  Value=x_qd
  Constant_x_qd_ab05a : Constant  Value=x_qd
  Constant_x_qd_b4ce8 : Constant  Value=x_qd
  Constant_x_qd_c1129 : Constant  Value=x_qd
  Constant_x_qd_c54cf : Constant  Value=x_qd
  Constant_x_qd_ceb2c : Constant  Value=x_qd
  Constant_x_qdd_1abcc : Constant  Value=x_qdd
  Constant_x_qdd_70164 : Constant  Value=x_qdd
  Constant_x_qdd_77313 : Constant  Value=x_qdd
  Constant_x_qdd_94532 : Constant  Value=x_qdd
  Constant_x_qdd_94e93 : Constant  Value=x_qdd
  Constant_x_qdd_bba48 : Constant  Value=x_qdd
  Constant_x_qdd_e5453 : Constant  Value=x_qdd
  Divide_035aa : Product  Inputs=*/
  Divide_1781f : Product  Inputs=*/
  Divide_3e200 : Product  Inputs=*/
  Divide_57b2c : Product  Inputs=*/
  Divide_a02bd : Product  Inputs=*/
  Divide_a34a6 : Product  Inputs=*/
  Divide_c9ea2 : Product  Inputs=*/
  Divide_f7d08 : Product  Inputs=*/
  Power_63d1b : Math  Operator=pow
  Product_19fd7 : Product
  Product_2a63b : Product
  Product_3fb95 : Product
  Product_4115a : Product
  Product_445c6 : Product
  Product_47eb0 : Product
  Product_5355b : Product
  Product_5baff : Product
  Product_64d63 : Product
  Product_a246f : Product
  Product_a48f1 : Product
  Product_bdd37 : Product
  Product_c00a7 : Product
  Product_ca425 : Product
  Product_e8c16 : Product
  Product_efb6b : Product
  Product_f5946 : Product
  Subtract_2c340 : Sum  Inputs=+-
  Subtract_545e2 : Sum  Inputs=+-
  Subtract_54976 : Sum  Inputs=+-
  Subtract_7131c : Sum  Inputs=+-
  Subtract_83592 : Sum  Inputs=+-
  Subtract_91326 : Sum  Inputs=+-
  Subtract_9e18b : Sum  Inputs=+-
  Subtract_f7d89 : Sum  Inputs=+-
  Blockout_d_psi_gq_SG_D_2_5c396 : Outport
  wires:
  Constant_x_l_1cdb8/1 -> Product_a48f1/2
  Constant_x_l_94af0/1 -> Product_f5946/2
  Constant_x_qd_65f47/1 -> Subtract_2c340/1
  Constant_x_l_a5099/1 -> Product_5355b/2
  Constant_x_qdd_94532/1 -> Subtract_f7d89/2
  Constant_-1_7b909/1 -> Product_2a63b/1
  Constant_-1_f5685/1 -> Product_19fd7/1
  State_psi_gq_SG_D_2_60145/1 -> Add_53508/1
  Constant_x_qdd_bba48/1 -> Subtract_2c340/2
  Constant_x_qd_ceb2c/1 -> Subtract_f7d89/1
  Constant_x_l_ff1cf/1 -> Product_2a63b/2
  Constant_x_l_301dc/1 -> Product_19fd7/2
  Product_2a63b/1 -> Add_8b7f8/1
  Product_19fd7/1 -> Add_a06be/1
  Constant_x_l_1d0ad/1 -> Product_a246f/2
  Constant_x_l_d8ef9/1 -> Product_4115a/2
  Constant_x_qd_c1129/1 -> Add_8b7f8/2
  Constant_x_qdd_94e93/1 -> Add_a06be/2
  Constant_-1_ac049/1 -> Product_a246f/1
  Constant_x_qd_0d74e/1 -> Add_6a6ac/2
  Constant_x_qdd_77313/1 -> Add_1961e/2
  State_psi_gq_SG_D_2_262a5/1 -> Product_445c6/1
  Add_8b7f8/1 -> Divide_035aa/2
  Add_a06be/1 -> Product_445c6/2
  Constant_x_qd_18b84/1 -> Subtract_545e2/2
  Product_a246f/1 -> Add_e2737/1
  Constant_x_qd_85f89/1 -> Add_e2737/2
  State_psi_kq_SG_D_2_b8dc9/1 -> Product_64d63/1
  Divide_a02bd/1 -> Subtract_7131c/1
  Subtract_2c340/1 -> Product_64d63/2
  Product_445c6/1 -> Divide_a02bd/1
  Add_e2737/1 -> Divide_a02bd/2
  Add_ea5d3/1 -> Product_bdd37/2
  Product_64d63/1 -> Divide_035aa/1
  Constant_-1_2b76b/1 -> Product_4115a/1
  Divide_035aa/1 -> Subtract_7131c/2
  Constant_-1_793ed/1 -> Product_a48f1/1
  Constant_-1_4cbd7/1 -> Product_f5946/1
  Product_4115a/1 -> Add_42289/1
  Constant_x_qdd_70164/1 -> Subtract_83592/2
  Constant_x_qd_b4ce8/1 -> Add_42289/2
  Subtract_7131c/1 -> Add_ea5d3/1
  Constant_-1_deea5/1 -> Product_5355b/1
  State_psi_q_SG_D_2_42d41/1 -> Add_ea5d3/2
  Product_a48f1/1 -> Add_6a6ac/1
  Product_f5946/1 -> Add_1961e/1
  Constant_-1_da27c/1 -> Product_efb6b/1
  Product_bdd37/1 -> Divide_a34a6/1
  Constant_x_l_f2337/1 -> Product_efb6b/2
  Product_3fb95/1 -> Add_9e869/2
  Constant_x_qd_ab05a/1 -> Subtract_83592/1
  Add_42289/1 -> Product_bdd37/1
  State_psi_gq_SG_D_2_d38f4/1 -> Product_5baff/1
  Add_6a6ac/1 -> Divide_f7d08/2
  Add_1961e/1 -> Product_5baff/2
  Product_efb6b/1 -> Add_a0dd7/1
  Constant_x_qd_c54cf/1 -> Add_a0dd7/2
  State_psi_kq_SG_D_2_bcc03/1 -> Product_c00a7/1
  Subtract_83592/1 -> Product_c00a7/2
  Divide_f7d08/1 -> Subtract_9e18b/2
  State_psi_kq_SG_D_2_628c0/1 -> Add_53508/2
  Product_c00a7/1 -> Divide_f7d08/1
  Constant_x_qdd_1abcc/1 -> Divide_a34a6/2
  Product_5baff/1 -> Divide_3e200/1
  Add_a0dd7/1 -> Divide_3e200/2
  Constant_-1_cc53b/1 -> Product_ca425/1
  Subtract_f7d89/1 -> Product_ca425/2
  Add_53508/1 -> Subtract_91326/1
  Divide_a34a6/1 -> Subtract_91326/2
  Product_5355b/1 -> Add_7d558/1
  Constant_x_qd_68c61/1 -> Add_7d558/2
  Divide_3e200/1 -> Subtract_9e18b/1
  Product_ca425/1 -> Product_47eb0/1
  Subtract_91326/1 -> Product_47eb0/2
  Add_7d558/1 -> Power_63d1b/1
  Constant_2.0_f9076/1 -> Power_63d1b/2
  Subtract_9e18b/1 -> Add_1aa89/1
  State_psi_q_SG_D_2_df93d/1 -> Add_1aa89/2
  Product_47eb0/1 -> Divide_57b2c/1
  Power_63d1b/1 -> Divide_57b2c/2
  Add_1aa89/1 -> Divide_1781f/1
  Constant_x_qdd_e5453/1 -> Divide_1781f/2
  Constant_x_q_8dd44/1 -> Subtract_545e2/1
  Divide_57b2c/1 -> Subtract_54976/1
  Divide_1781f/1 -> Subtract_54976/2
  Divide_c9ea2/1 -> Blockout_d_psi_gq_SG_D_2_5c396/1
  Constant_-1_2ef28/1 -> Product_e8c16/1
  State_psi_gq_SG_D_2_ab3da/1 -> Product_e8c16/2
  Subtract_545e2/1 -> Product_3fb95/1
  Subtract_54976/1 -> Product_3fb95/2
  Product_e8c16/1 -> Add_9e869/1
  Add_9e869/1 -> Divide_c9ea2/1
  Constant_T_qd_efd98/1 -> Divide_c9ea2/2

== system case4/SG_D_2/d_psi_kq_SG_D_2_block ==
  note: d_psi_kq_SG_D_2 in case4
      | $-\frac{\psi _{\mathrm{gq},\mathrm{SG},D,2}+\psi _{\mathrm{kq},\mathrm{SG},D,2}+\frac{\left(x_{l}-x_{\mathrm{qd}}\right)\,\left(\psi _{q,\mathrm{SG},D,2}+\frac{\psi _{\mathrm{gq},\mathrm{SG},D,2}\,\left(x_{l}-x_{\mathrm{qdd}}\right)}{x_{l}-x_{\mathrm{qd}}}+\frac{\psi _{\mathrm{kq},\mathrm{SG},D,2}\,\left(x_{\mathrm{qd}}-x_{\mathrm{qdd}}\right)}{x_{l}-x_{\mathrm{qd}}}\right)}{x_{\mathrm{qdd}}}}{T_{\mathrm{qdd}}}$
      | Automatically generated on 2025-10-31 19:05:32 .
  State_psi_gq_SG_D_2_8d7c7 : Inport
  State_psi_kq_SG_D_2_02eb9 : Inport  Port=2
  State_psi_gq_SG_D_2_77eb3 : Inport  Port=3
  State_psi_kq_SG_D_2_92652 : Inport  Port=4
  State_psi_q_SG_D_2_06ac6 : Inport  Port=5
  Add_1f8ec : Sum
  Add_6a030 : Sum
  Add_6fe76 : Sum
  Add_87ad2 : Sum
  Add_9fa4e : Sum
  Add_ed996 : Sum
  Constant_-1_5785f : Constant  Value=-1
  Constant_-1_5ec3d : Constant  Value=-1
  Constant_-1_66d0a : Constant  Value=-1
  Constant_-1_7705c : Constant  Value=-1
  Constant_-1_f8176 : Constant  Value=-1
  Constant_T_qdd_dd080 : Constant  Value=T_qdd
  Constant_x_l_55f72 : Constant  Value=x_l
  Constant_x_l_61762 : Constant  Value=x_l
  Constant_x_l_74e4e : Constant  Value=x_l
  Constant_x_l_de384 : Constant  Value=x_l
  Constant_x_qd_1e6d6 : Constant  Value=x_qd
  Constant_x_qd_41fc8 : Constant  Value=x_qd
  Constant_x_qd_c5760 : Constant  Value=x_qd
  Constant_x_qd_d905b : Constant  Value=x_qd
  Constant_x_qdd_471f4 : Constant  Value=x_qdd
  Constant_x_qdd_cc495 : Constant  Value=x_qdd
  Constant_x_qdd_eb158 : Constant  Value=x_qdd
  Divide_3461c : Product  Inputs=*/
  Divide_4f83f : Product  Inputs=*/
  Divide_aa5f1 : Product  Inputs=*/
  Divide_c1a86 : Product  Inputs=*/
  Product_17c94 : Product
  Product_410ab : Product
  Product_82bca : Product
  Product_873e3 : Product
  Product_bfabc : Product
  Product_ce151 : Product
  Product_e69de : Product
  Product_e8785 : Product
  Subtract_048f9 : Sum  Inputs=+-
  Subtract_6d652 : Sum  Inputs=+-
  Subtract_7123f : Sum  Inputs=+-
  Blockout_d_psi_kq_SG_D_2_5a47a : Outport
  wires:
  State_psi_kq_SG_D_2_02eb9/1 -> Subtract_7123f/2
  Constant_-1_7705c/1 -> Product_17c94/1
  Constant_-1_66d0a/1 -> Product_410ab/1
  Constant_x_l_de384/1 -> Product_410ab/2
  Constant_x_qdd_eb158/1 -> Add_9fa4e/2
  Constant_x_l_61762/1 -> Product_17c94/2
  Constant_x_qd_41fc8/1 -> Subtract_6d652/1
  Constant_T_qdd_dd080/1 -> Divide_c1a86/2
  Constant_-1_5785f/1 -> Product_e69de/1
  Product_410ab/1 -> Add_9fa4e/1
  Constant_x_qdd_cc495/1 -> Subtract_6d652/2
  Constant_x_l_74e4e/1 -> Product_e69de/2
  Divide_c1a86/1 -> Blockout_d_psi_kq_SG_D_2_5a47a/1
  State_psi_gq_SG_D_2_77eb3/1 -> Product_82bca/1
  Add_9fa4e/1 -> Product_82bca/2
  Product_17c94/1 -> Add_1f8ec/1
  Constant_x_qd_1e6d6/1 -> Add_1f8ec/2
  Product_bfabc/1 -> Divide_aa5f1/1
  State_psi_kq_SG_D_2_92652/1 -> Product_e8785/1
  Subtract_6d652/1 -> Product_e8785/2
  Product_e69de/1 -> Add_6fe76/1
  Constant_x_qd_d905b/1 -> Add_6fe76/2
  Product_e8785/1 -> Divide_4f83f/1
  Product_82bca/1 -> Divide_3461c/1
  Add_1f8ec/1 -> Divide_3461c/2
  Add_6fe76/1 -> Divide_4f83f/2
  State_psi_q_SG_D_2_06ac6/1 -> Add_6a030/2
  Constant_-1_f8176/1 -> Product_ce151/1
  Constant_x_l_55f72/1 -> Product_ce151/2
  Divide_3461c/1 -> Subtract_048f9/1
  Divide_4f83f/1 -> Subtract_048f9/2
  Product_ce151/1 -> Add_ed996/1
  Constant_x_qd_c5760/1 -> Add_ed996/2
  Subtract_048f9/1 -> Add_6a030/1
  Constant_x_qdd_471f4/1 -> Divide_aa5f1/2
  Constant_-1_5ec3d/1 -> Product_873e3/1
  State_psi_gq_SG_D_2_8d7c7/1 -> Product_873e3/2
  Add_ed996/1 -> Product_bfabc/1
  Add_6a030/1 -> Product_bfabc/2
  Product_873e3/1 -> Subtract_7123f/1
  Subtract_7123f/1 -> Add_87ad2/1
  Divide_aa5f1/1 -> Add_87ad2/2
  Add_87ad2/1 -> Divide_c1a86/1

== system case4/SG_D_2/d_psi_q_SG_D_2_block ==
  note: d_psi_q_SG_D_2 in case4
      | $2\,\pi \,f_{0}\,\left(v_{d,\mathrm{SG},D,2}\,\cos\left(\theta _{\mathrm{SG},D,2}\right)+v_{q,\mathrm{SG},D,2}\,\sin\left(\theta _{\mathrm{SG},D,2}\right)-\frac{R_{a}\,\left(\psi _{q,\mathrm{SG},D,2}+\frac{\psi _{\mathrm{gq},\mathrm{SG},D,2}\,\left(x_{l}-x_{\mathrm{qdd}}\right)}{x_{l}-x_{\mathrm{qd}}}+\frac{\psi _{\mathrm{kq},\mathrm{SG},D,2}\,\left(x_{\mathrm{qd}}-x_{\mathrm{qdd}}\right)}{x_{l}-x_{\mathrm{qd}}}\right)}{x_{\mathrm{qdd}}}-\frac{\psi _{d,\mathrm{SG},D,2}\,w_{\mathrm{SG},D,2}}{2\,f_{0}\,\pi }\right)$
      | Automatically generated on 2025-10-31 19:05:17 .
  State_psi_gq_SG_D_2_e6c3e : Inport
  State_psi_kq_SG_D_2_849d4 : Inport  Port=2
  State_psi_q_SG_D_2_7ccc9 : Inport  Port=3
  Input_v_d_SG_D_2_9a544 : Inport  Port=4
  State_theta_SG_D_2_14fc9 : Inport  Port=5
  Input_v_q_SG_D_2_bd14d : Inport  Port=6
  State_theta_SG_D_2_47b3e : Inport  Port=7
  State_psi_d_SG_D_2_a9787 : Inport  Port=8
  State_w_SG_D_2_85500 : Inport  Port=9
  Add_0cd5b : Sum
  Add_30634 : Sum
  Add_616a5 : Sum
  Add_653bc : Sum
  Add_b44b2 : Sum
  Constant_-1_3241b : Constant  Value=-1
  Constant_-1_8a237 : Constant  Value=-1
  Constant_-1_bd3ff : Constant  Value=-1
  Constant_-2.0_d78db : Constant  Value=-2.0
  Constant_2.0_14661 : Constant  Value=2.0
  Constant_R_a_83cc8 : Constant  Value=R_a
  Constant_f0_455ab : Constant  Value=f0
  Constant_f0_f1981 : Constant  Value=f0
  Constant_pi_2f37a : Constant  Value=pi
  Constant_pi_4c847 : Constant  Value=pi
  Constant_x_l_1b278 : Constant  Value=x_l
  Constant_x_l_71e2c : Constant  Value=x_l
  Constant_x_l_9724a : Constant  Value=x_l
  Constant_x_qd_0316c : Constant  Value=x_qd
  Constant_x_qd_642fe : Constant  Value=x_qd
  Constant_x_qd_8c883 : Constant  Value=x_qd
  Constant_x_qdd_21873 : Constant  Value=x_qdd
  Constant_x_qdd_93bc1 : Constant  Value=x_qdd
  Constant_x_qdd_cd977 : Constant  Value=x_qdd
  Divide_7705b : Product  Inputs=*/
  Divide_8763b : Product  Inputs=*/
  Divide_a6b1e : Product  Inputs=*/
  Divide_e29bf : Product  Inputs=*/
  MathFunc_cos_a1dcf : Trigonometry  Operator=cos
  MathFunc_sin_846fe : Trigonometry
  Product_15606 : Product
  Product_2dedc : Product
  Product_33894 : Product
  Product_47d42 : Product
  Product_58a5f : Product
  Product_5eda7 : Product
  Product_68a9d : Product
  Product_77242 : Product
  Product_9a1ca : Product
  Product_a669b : Product
  Product_a76bb : Product
  Product_b693a : Product
  Product_d863c : Product
  Product_f0b9e : Product
  Subtract_2728c : Sum  Inputs=+-
  Subtract_8cc88 : Sum  Inputs=+-
  Subtract_9444f : Sum  Inputs=+-
  Subtract_c85ef : Sum  Inputs=+-
  Blockout_d_psi_q_SG_D_2_4e8af : Outport
  wires:
  Constant_x_qdd_93bc1/1 -> Subtract_2728c/2
  Constant_x_l_1b278/1 -> Product_a669b/2
  Constant_-1_8a237/1 -> Product_2dedc/1
  Constant_x_l_9724a/1 -> Product_2dedc/2
  Product_2dedc/1 -> Add_b44b2/1
  Constant_pi_2f37a/1 -> Product_15606/2
  State_psi_gq_SG_D_2_e6c3e/1 -> Product_58a5f/1
  Constant_x_l_71e2c/1 -> Product_9a1ca/2
  State_w_SG_D_2_85500/1 -> Product_d863c/2
  Constant_x_qd_0316c/1 -> Add_30634/2
  Constant_x_qdd_cd977/1 -> Add_b44b2/2
  Constant_2.0_14661/1 -> Product_15606/1
  Constant_-1_bd3ff/1 -> Product_9a1ca/1
  Constant_x_qd_642fe/1 -> Subtract_2728c/1
  Constant_-1_3241b/1 -> Product_a669b/1
  State_psi_q_SG_D_2_7ccc9/1 -> Add_616a5/2
  Add_b44b2/1 -> Product_58a5f/2
  Product_15606/1 -> Product_a76bb/1
  Product_9a1ca/1 -> Add_0cd5b/1
  Constant_pi_4c847/1 -> Product_f0b9e/2
  Constant_f0_455ab/1 -> Product_a76bb/2
  Constant_x_qd_8c883/1 -> Add_0cd5b/2
  State_psi_kq_SG_D_2_849d4/1 -> Product_b693a/1
  Subtract_2728c/1 -> Product_b693a/2
  Product_a669b/1 -> Add_30634/1
  Input_v_q_SG_D_2_bd14d/1 -> Product_33894/1
  Product_58a5f/1 -> Divide_a6b1e/1
  Product_a76bb/1 -> Divide_e29bf/2
  Add_0cd5b/1 -> Divide_a6b1e/2
  Product_b693a/1 -> Divide_7705b/1
  Add_30634/1 -> Divide_7705b/2
  Divide_a6b1e/1 -> Subtract_c85ef/1
  State_theta_SG_D_2_14fc9/1 -> MathFunc_cos_a1dcf/1
  Divide_7705b/1 -> Subtract_c85ef/2
  Subtract_c85ef/1 -> Add_616a5/1
  MathFunc_cos_a1dcf/1 -> Product_77242/2
  Constant_R_a_83cc8/1 -> Product_47d42/1
  Add_616a5/1 -> Product_47d42/2
  State_theta_SG_D_2_47b3e/1 -> MathFunc_sin_846fe/1
  Product_47d42/1 -> Divide_8763b/1
  Product_f0b9e/1 -> Product_68a9d/1
  Product_33894/1 -> Subtract_9444f/2
  Constant_x_qdd_21873/1 -> Divide_8763b/2
  Input_v_d_SG_D_2_9a544/1 -> Product_77242/1
  Add_653bc/1 -> Product_5eda7/2
  Divide_8763b/1 -> Subtract_8cc88/1
  Product_77242/1 -> Subtract_8cc88/2
  MathFunc_sin_846fe/1 -> Product_33894/2
  Product_5eda7/1 -> Blockout_d_psi_q_SG_D_2_4e8af/1
  State_psi_d_SG_D_2_a9787/1 -> Product_d863c/1
  Constant_-2.0_d78db/1 -> Product_f0b9e/1
  Product_68a9d/1 -> Product_5eda7/1
  Subtract_8cc88/1 -> Subtract_9444f/1
  Product_d863c/1 -> Divide_e29bf/1
  Constant_f0_f1981/1 -> Product_68a9d/2
  Subtract_9444f/1 -> Add_653bc/1
  Divide_e29bf/1 -> Add_653bc/2

== system case4/SG_D_2/d_theta_SG_D_2_block ==
  note: d_theta_SG_D_2 in case4
      | $w_{\mathrm{SG},D,2}-2\,\pi \,f_{0}$
      | Automatically generated on 2025-10-31 19:05:39 .
  State_w_SG_D_2_83554 : Inport
  Add_7e58a : Sum
  Constant_-2.0_bfc3a : Constant  Value=-2.0
  Constant_f0_9b662 : Constant  Value=f0
  Constant_pi_7f438 : Constant  Value=pi
  Product_72dcc : Product
  Product_a418d : Product
  Blockout_d_theta_SG_D_2_36a6f : Outport
  wires:
  Constant_-2.0_bfc3a/1 -> Product_a418d/1
  Constant_pi_7f438/1 -> Product_a418d/2
  Add_7e58a/1 -> Blockout_d_theta_SG_D_2_36a6f/1
  Product_a418d/1 -> Product_72dcc/1
  Constant_f0_9b662/1 -> Product_72dcc/2
  Product_72dcc/1 -> Add_7e58a/1
  State_w_SG_D_2_83554/1 -> Add_7e58a/2
